simulink model "asm1_w_settler"  (R2023b)
settings: Solver=ode15s  StartTime=0.0  StopTime=200  FixedStep=0.01  RelTol=1e-5  AbsTol=1e-8
undefined symbols (not defined in the file): ACTIVATE, DIM, LAYER, MODELTYPE, PAR1, Qr, Qw, SETTLERINIT, SETTLERPAR, T, TEMPMODEL, XINITDELAYPRIMARY
settings Model: Creator=ielulf  LastModifiedBy=BuB
settings SolverCC: AutoScaleAbsTol=off  AlgebraicLoopSolver=TrustRegion
settings DataIOCC: InitialState=xFinal  SaveFormat=Array  SignalLoggingSaveFormat=ModelDataLogs  SaveOutput=off  ReturnWorkspaceOutputs=off  TimeSaveName=t  SignalLoggingName=sigsOut  OutputTimes=[0:(1/96):609]
settings OptimizationCC: BlockReduction=off  BooleanDataType=off  OptimizeBlockIOStorage=off  BufferReuse=off  GlobalBufferReuse=off  ExpressionFolding=off  LocalBlockOutputs=off  InitFltsAndDblsToZero=on  LifeSpan=inf  OptimizeDataStoreBuffers=off  BusAssignmentInplaceUpdate=off
settings DebuggingCC: SaveWithParameterizedLinksMsg=none  UnderspecifiedInitializationDetection=Classic  MergeDetectMultiDrivingBlocksExec=none  SignalResolutionControl=TryResolveAllWithWarning  InheritedTsInSrcMsg=none  MultiTaskDSMMsg=warning  MultiTaskCondExecSysMsg=none  FcnCallInpInsideContextMsg=warning  UnconnectedInputMsg=warning  UnconnectedLineMsg=warning  SFUnexpectedBacktrackingDiag=warning  SFNoUnconditionalDefaultTransitionDiag=warning  SFExecutionAtInitializationDiag=none  ArithmeticOperatorsInVariantConditions=warning
settings HardwareCC: ProdBitPerPointer=32  ProdBitPerSizeT=32  ProdBitPerPtrDiffT=32  ProdLargestAtomicFloat=None  ProdIntDivRoundTo=Undefined  ProdEndianess=Unspecified  ProdWordSize=32  ProdHWDeviceType=32-bit Generic  TargetUnknown=on
settings ModelReferenceCC: EnableRefExpFcnMdlSchedulingChecks=on  PropagateSignalLabelsOutOfModel=off
settings RTWCC: TemplateMakefile=grt_unix.tmf
settings CodeAppCC: StateflowObjectComments=on
settings GRTTargetCC: TargetFcnLib=ansi_tfl_tmw.mat  TargetLangStandard=C89/C90 (ANSI)  CombineOutputUpdateFcns=off  GRTInterface=on
settings ConfigComp: CovMetricSettings=dw  CovSaveCumulativeToWorkspaceVar=on  CovSaveSingleToWorkspaceVar=on

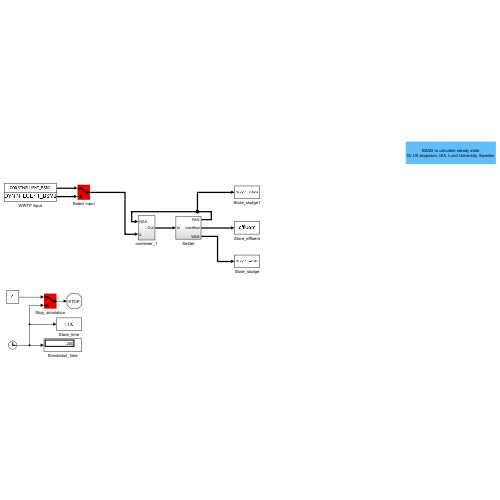
[thumbnail: Simulink's stored preview of the top-level diagram]
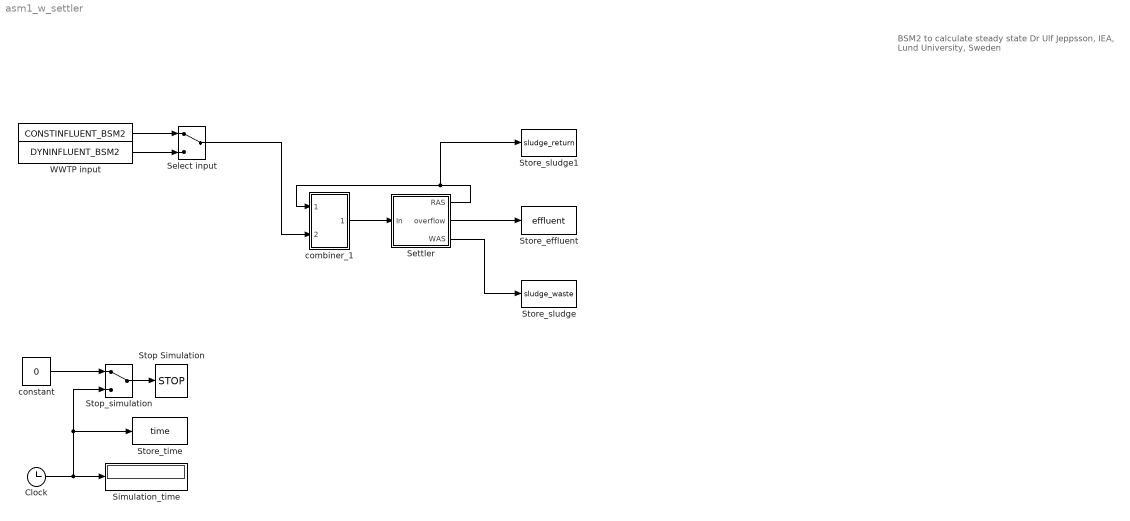
== system asm1_w_settler ==
  note: BSM2 to calculate steady state
      |  Dr Ulf Jeppsson, IEA, Lund University, Sweden
  " " : FromWorkspace  VariableName=CONSTINFLUENT_BSM2  SampleTime=-1  ZeroCross=off  OutputAfterFinalValue=Holding final value
  " constant" : Constant  Value=0
  Clock : Clock
  Select input : ManualSwitch
  Settler : Subsystem
  Simulation_time : Display
  Stop Simulation : Stop
  Stop_simulation : ManualSwitch
  Store_effluent : ToWorkspace  VariableName=effluent
  Store_sludge : ToWorkspace  VariableName=sludge_waste
  Store_sludge1 : ToWorkspace  VariableName=sludge_return
  Store_time : ToWorkspace  VariableName=time
  WWTP input : FromWorkspace  VariableName=DYNINFLUENT_BSM2  SampleTime=-1  ZeroCross=off  OutputAfterFinalValue=Holding final value
  combiner_1 : Subsystem
  wires:
  Settler/3(WAS) -> Store_sludge/1
  Settler/2(overflow) -> Store_effluent/1
  Clock/1 -> Simulation_time/1, Stop_simulation/2, Store_time/1
  Stop_simulation/1 -> Stop Simulation/1
  " constant"/1 -> Stop_simulation/1
  Select input/1 -> combiner_1/2(In2)
  " "/1 -> Select input/1
  WWTP input/1 -> Select input/2
  Settler/1(RAS) -> Store_sludge1/1, combiner_1/1(RAS)
  combiner_1/1(Out) -> Settler/1(In)

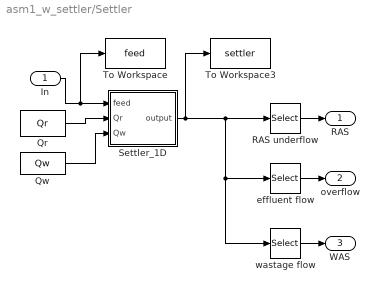
== system asm1_w_settler/Settler ==
  In : Inport
  Qr : Constant  Value=Qr
  Qw : Constant  Value=Qw
  RAS underflow : Selector  InputPortWidth=166  IndexOptions=Index vector (dialog)  Indices=[1:21]  OutputSizes=1
  Settler_1D : Subsystem
  To Workspace : ToWorkspace  VariableName=feed
  To Workspace3 : ToWorkspace  VariableName=settler
  effluent flow : Selector  InputPortWidth=166  IndexOptions=Index vector (dialog)  Indices=[23:43]  OutputSizes=1
  wastage flow : Selector  InputPortWidth=166  IndexOptions=Index vector (dialog)  Indices=[1:14,22,16:21]  OutputSizes=1
  RAS : Outport
  overflow : Outport  Port=2
  WAS : Outport  Port=3
  wires:
  In/1 -> To Workspace/1, Settler_1D/1(feed)
  Settler_1D/1(output) -> RAS underflow/1, effluent flow/1, wastage flow/1, To Workspace3/1
  wastage flow/1 -> WAS/1
  effluent flow/1 -> overflow/1
  RAS underflow/1 -> RAS/1
  Qr/1 -> Settler_1D/2(Qr)
  Qw/1 -> Settler_1D/3(Qw)

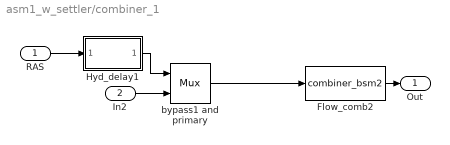
== system asm1_w_settler/combiner_1 ==
  RAS : Inport
  In2 : Inport  Port=2
  Flow_comb2 : S-Function  FunctionName=combiner_bsm2  SFunctionDeploymentMode=off  EnableBusSupport=off
  Hyd_delay1 : Subsystem
  bypass1 and primary : Mux  Inputs=2
  Out : Outport
  wires:
  RAS/1 -> Hyd_delay1/1(Input)
  Flow_comb2/1 -> Out/1
  In2/1 -> bypass1 and primary/2
  bypass1 and primary/1 -> Flow_comb2/1
  Hyd_delay1/1(Output) -> bypass1 and primary/1

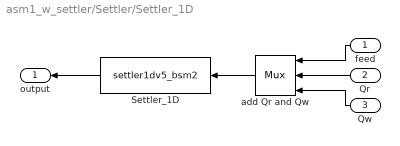
== system asm1_w_settler/Settler/Settler_1D ==
  feed : Inport
  Qr : Inport  Port=2
  Qw : Inport  Port=3
  Settler_1D : S-Function  FunctionName=settler1dv5_bsm2  Parameters=SETTLERINIT,SETTLERPAR,DIM,LAYER,MODELTYPE,TEMPMODEL,ACTIVATE  SFunctionDeploymentMode=off  EnableBusSupport=off
  add Qr and Qw : Mux  Inputs=3
  output : Outport
  wires:
  Settler_1D/1 -> output/1
  feed/1 -> add Qr and Qw/1
  Qw/1 -> add Qr and Qw/3
  Qr/1 -> add Qr and Qw/2
  add Qr and Qw/1 -> Settler_1D/1

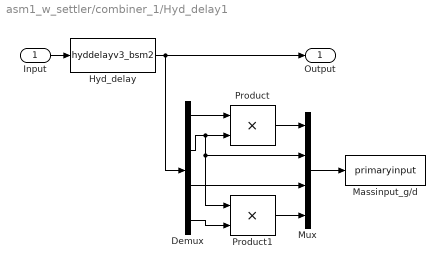
== system asm1_w_settler/combiner_1/Hyd_delay1 ==
  Input : Inport
  Demux : Demux  Outputs=[14,1,1,5]
      settings: DisplayOption=none
  Hyd_delay : S-Function  FunctionName=hyddelayv3_bsm2  Parameters=XINITDELAYPRIMARY,PAR1,T  SFunctionDeploymentMode=off  EnableBusSupport=off
  Massinput_g/d : ToWorkspace  VariableName=primaryinput  SampleTime=-1
  Mux : Mux
  Product : Product  SaturateOnIntegerOverflow=on  OutDataTypeStr=Inherit: Same as first input
  Product1 : Product  SaturateOnIntegerOverflow=on  OutDataTypeStr=Inherit: Same as first input
  Output : Outport
  wires:
  Demux/4 -> Product1/2
  Product1/1 -> Mux/4
  Demux/3 -> Mux/3
  Demux/2 -> Product1/1, Mux/2, Product/2
  Input/1 -> Hyd_delay/1
  Hyd_delay/1 -> Demux/1, Output/1
  Demux/1 -> Product/1
  Product/1 -> Mux/1
  Mux/1 -> Massinput_g/d/1
